simulink model "HEARTVI110"  (Simulink 5.0)
settings: Solver=ode45  StartTime=0.0  StopTime=3  RelTol=1e-3
libraries: simulink x3
settings Model: Creator=Dit Papa Lamine NDao  LastModifiedBy=formateur  SaveTime=off  SaveOutput=off  LimitDataPoints=off

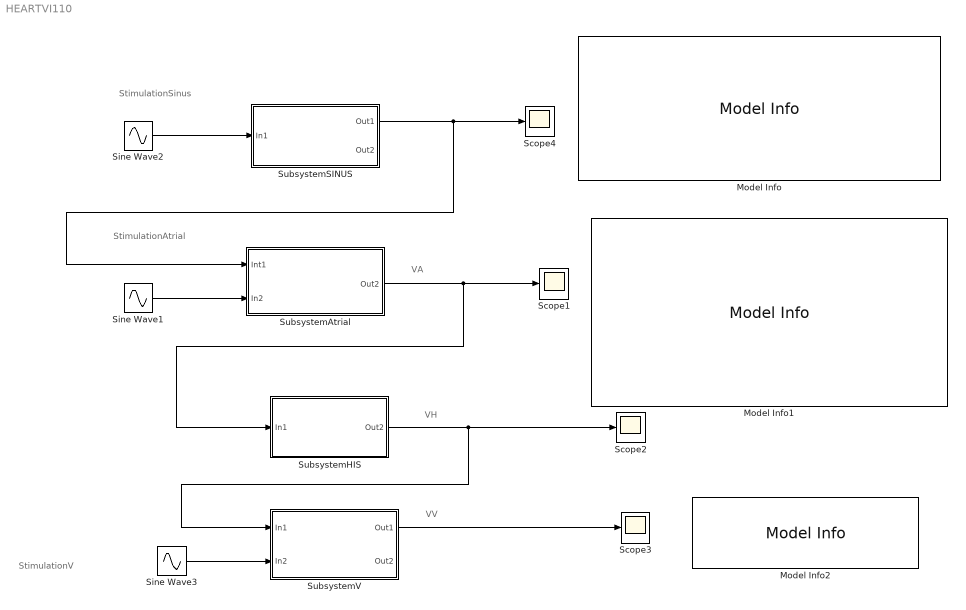
== system HEARTVI110 ==
  note: StimulationSinus
  note: StimulationAtrial
  note: VA
  note: VH
  note: VV
  note: StimulationV
  Model Info : simulink/Model-Wide Utilities/Model Info  InitialBlockCM=None  BlockCM=None  Frame=on  DisplayStringWithTags=|  HorizontalTextAlignment=Center  LeftAlignmentValue=0.5  SourceBlockDiagram=HEARTVI110  TagMaxNumber=20
      | NEW BLOCK LIBRARY SIMULINK
      | BLOCK HEART VI
      | TUTORIAL BY DIT.P.L.NDAO
      | BUREAU EA dakar senegal
      | www.cardiorythmor-vibrator.com
      | TUTORIAL N°1 date 8/12/2009
      | patants ndao france 2005
      | copyright ndao 2007
  Model Info1 : simulink/Model-Wide Utilities/Model Info  InitialBlockCM=None  BlockCM=None  Frame=on  DisplayStringWithTags=|  HorizontalTextAlignment=Center  LeftAlignmentValue=0.5  SourceBlockDiagram=HEARTVI110  TagMaxNumber=20
      | INVESTIGATION WITH HEART VI1
      | 1)I begin with no normal heart beating 
      | Fs=2Fa=2Fv
      | 2)i change parameter sinus and
      |  i publish annihilation of heart rythm past days.
      | 3)I Re-Synchronize the heart beat i
      | n this case.
      | of no normal heart beating.
      | Rational cardiac parameters.
      | Stimulation of normal sinus rythm of sinus,that 
      | induces Polymorphic Arrythmias like Wakenbach Syndrom-Sinusal Stimulation means Central
      | nervous reaction---Input stimulation Asinwt
      | A=2  w=2
  Model Info2 : simulink/Model-Wide Utilities/Model Info  InitialBlockCM=None  BlockCM=None  Frame=on  DisplayStringWithTags=|  HorizontalTextAlignment=Center  LeftAlignmentValue=0.5  SourceBlockDiagram=HEARTVI110  TagMaxNumber=20
      | DATE;7/01/2010
      | -Sinusal stimulation of a normal sinus rythm
      | -Duration of computing:4mn
  Scope{1..4} (4 alike) : Scope
      Scope1 settings: YMin=-2  YMax=2  SaveName=ScopeData3
      Scope2 settings: YMin=-2  YMax=2  SaveName=ScopeData4
      Scope3 settings: YMin=-2  YMax=2  SaveName=ScopeData5
      Scope4 settings: YMin=-2  YMax=2  SaveName=ScopeData2
  Sine Wave1 : Sin  Amplitude=0  SampleTime=0
  Sine Wave2 : Sin  Amplitude=-206  Frequency=5  SampleTime=0
  Sine Wave3 : Sin  Amplitude=0  Frequency=2.4  SampleTime=0
  SubsystemAtrial : Subsystem
  SubsystemHIS : Subsystem
  SubsystemSINUS : Subsystem
  SubsystemV : Subsystem
  wires:
  SubsystemAtrial/1(Out2) -> Scope1/1, SubsystemHIS/1(In1)
  SubsystemHIS/1(Out2) -> Scope2/1, SubsystemV/1(In1)
  SubsystemV/1(Out1) -> Scope3/1
  Sine Wave2/1 -> SubsystemSINUS/1(In1)
  Sine Wave1/1 -> SubsystemAtrial/2(In2)
  Sine Wave3/1 -> SubsystemV/2(In2)
  SubsystemSINUS/1(Out1) -> SubsystemAtrial/1(Int1), Scope4/1

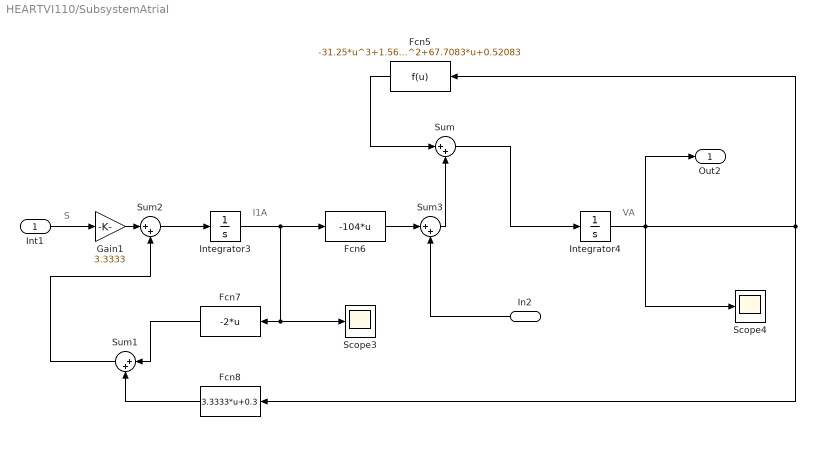
== system HEARTVI110/SubsystemAtrial ==
  note: I1A
  note: VA
  note: S
  Int1 : Inport  ShowAdditionalParam=on  DataType=double
  In2 : Inport  Orientation=left  Port=2
  Fcn5 : Fcn  Orientation=left  Expr=-31.25*u^3+1.5625*u^2+67.7083*u+0.52083
  Fcn6 : Fcn  Expr=-104*u
  Fcn7 : Fcn  Orientation=left  Expr=-2*u
  Fcn8 : Fcn  Orientation=left  Expr=3.3333*u+0.3
  Gain1 : Gain  Gain=3.3333  SaturateOnIntegerOverflow=on
  Integrator3 : Integrator  InitialCondition=0.00096  ZeroCross=off
  Integrator4 : Integrator  InitialCondition=-0.05  ZeroCross=off
  Scope3 : Scope
      settings: YMin=-2  YMax=2
  Scope4 : Scope
      settings: YMin=-2  YMax=2
  Sum : Sum  Inputs=|++  SaturateOnIntegerOverflow=on
  Sum1 : Sum  Orientation=left  Inputs=|++  SaturateOnIntegerOverflow=on
  Sum2 : Sum  Inputs=|++  SaturateOnIntegerOverflow=on
  Sum3 : Sum  Inputs=|++  SaturateOnIntegerOverflow=on
  Out2 : Outport
  wires:
  Fcn5/1 -> Sum/1
  Integrator3/1 -> Fcn6/1, Fcn7/1, Scope3/1
  Sum/1 -> Integrator4/1
  Integrator4/1 -> Fcn5/1, Fcn8/1, Scope4/1, Out2/1
  Fcn7/1 -> Sum1/1
  Fcn8/1 -> Sum1/2
  Fcn6/1 -> Sum3/1
  Sum3/1 -> Sum/2
  Int1/1 -> Gain1/1
  Gain1/1 -> Sum2/1
  Sum2/1 -> Integrator3/1
  Sum1/1 -> Sum2/2
  In2/1 -> Sum3/2

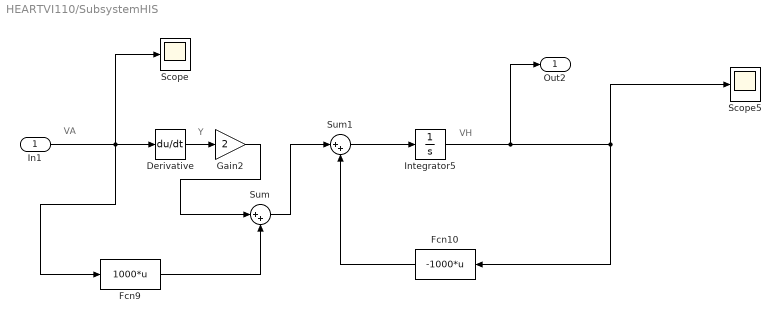
== system HEARTVI110/SubsystemHIS ==
  note: VH
  note: Y
  note: VA
  In1 : Inport  PortDimensions=159  ShowAdditionalParam=on  DataType=double
  Derivative : Derivative
  Fcn10 : Fcn  Orientation=left  Expr=-1000*u
  Fcn9 : Fcn  Expr=1000*u
  Gain2 : Gain  Gain=2  SaturateOnIntegerOverflow=on
  Integrator5 : Integrator  InitialCondition=-0.05  ZeroCross=off
  Scope : Scope
  Scope5 : Scope
      settings: YMin=-0.001  YMax=0.001
  Sum : Sum  Inputs=|++  SaturateOnIntegerOverflow=on
  Sum1 : Sum  Inputs=|++  SaturateOnIntegerOverflow=on
  Out2 : Outport
  wires:
  Integrator5/1 -> Fcn10/1, Scope5/1, Out2/1
  Fcn9/1 -> Sum/2
  Sum/1 -> Sum1/1
  Fcn10/1 -> Sum1/2
  Sum1/1 -> Integrator5/1
  Derivative/1 -> Gain2/1
  Gain2/1 -> Sum/1
  In1/1 -> Derivative/1, Scope/1, Fcn9/1

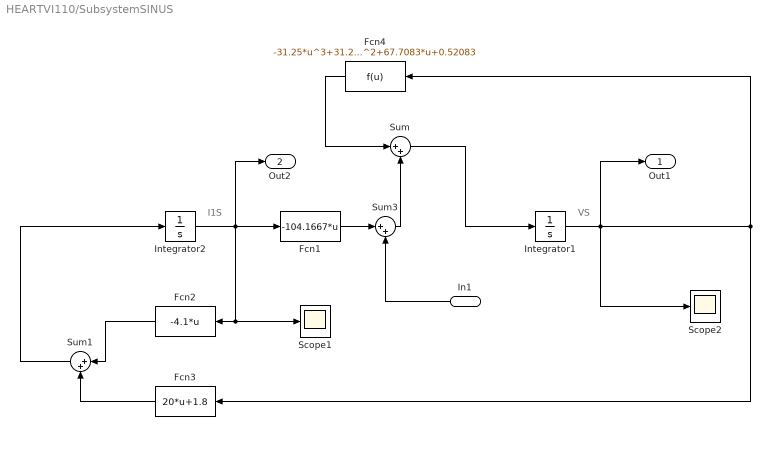
== system HEARTVI110/SubsystemSINUS ==
  note: I1S
  note: VS
  In1 : Inport  Orientation=left
  Fcn1 : Fcn  Expr=-104.1667*u
  Fcn2 : Fcn  Orientation=left  Expr=-4.1*u
  Fcn3 : Fcn  Orientation=left  Expr=20*u+1.8
  Fcn4 : Fcn  Orientation=left  Expr=-31.25*u^3+31.25*u^2+67.7083*u+0.52083
  Integrator1 : Integrator  InitialCondition=-0.05  ZeroCross=off
  Integrator2 : Integrator  InitialCondition=0.00096  ZeroCross=off
  Scope1 : Scope
      settings: YMin=-2  YMax=2
  Scope2 : Scope
      settings: YMin=-2  YMax=2
  Sum : Sum  Inputs=|++  SaturateOnIntegerOverflow=on
  Sum1 : Sum  Orientation=left  Inputs=|++  SaturateOnIntegerOverflow=on
  Sum3 : Sum  Inputs=|++  SaturateOnIntegerOverflow=on
  Out1 : Outport
  Out2 : Outport  Port=2
  wires:
  Fcn4/1 -> Sum/1
  Integrator2/1 -> Fcn1/1, Fcn2/1, Scope1/1, Out2/1
  Sum/1 -> Integrator1/1
  Integrator1/1 -> Fcn4/1, Fcn3/1, Scope2/1, Out1/1
  Fcn2/1 -> Sum1/1
  Fcn3/1 -> Sum1/2
  Fcn1/1 -> Sum3/1
  Sum3/1 -> Sum/2
  Sum1/1 -> Integrator2/1
  In1/1 -> Sum3/2

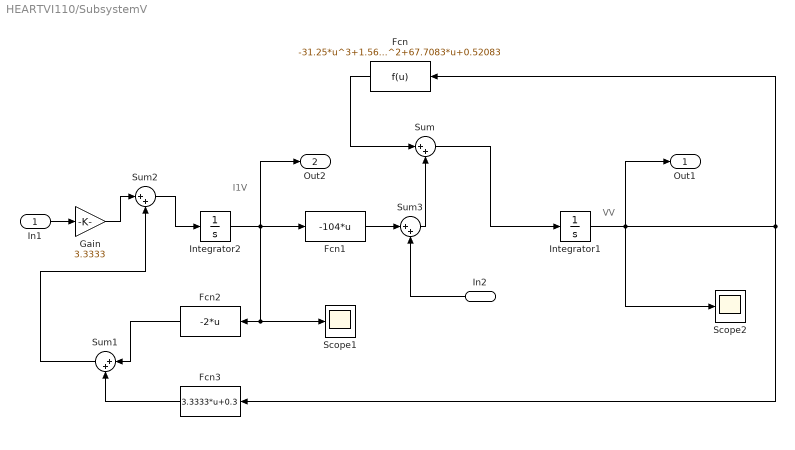
== system HEARTVI110/SubsystemV ==
  note: VV
  note: I1V
  In1 : Inport
  In2 : Inport  Orientation=left  Port=2
  Fcn : Fcn  Orientation=left  Expr=-31.25*u^3+1.5625*u^2+67.7083*u+0.52083
  Fcn1 : Fcn  Expr=-104*u
  Fcn2 : Fcn  Orientation=left  Expr=-2*u
  Fcn3 : Fcn  Orientation=left  Expr=3.3333*u+0.3
  Gain : Gain  Gain=3.3333  SaturateOnIntegerOverflow=on
  Integrator1 : Integrator  InitialCondition=-0.05  ZeroCross=off
  Integrator2 : Integrator  InitialCondition=0.00096  ZeroCross=off
  Scope1 : Scope
      settings: YMin=-2  YMax=2
  Scope2 : Scope
      settings: YMin=-2  YMax=2
  Sum : Sum  Inputs=|++  SaturateOnIntegerOverflow=on
  Sum1 : Sum  Orientation=left  Inputs=|++  SaturateOnIntegerOverflow=on
  Sum2 : Sum  Inputs=|++  SaturateOnIntegerOverflow=on
  Sum3 : Sum  Inputs=|++  SaturateOnIntegerOverflow=on
  Out1 : Outport
  Out2 : Outport  Port=2
  wires:
  In1/1 -> Gain/1
  In2/1 -> Sum3/2
  Sum1/1 -> Sum2/2
  Gain/1 -> Sum2/1
  Sum3/1 -> Sum/2
  Fcn1/1 -> Sum3/1
  Fcn3/1 -> Sum1/2
  Fcn2/1 -> Sum1/1
  Integrator1/1 -> Fcn/1, Fcn3/1, Out1/1, Scope2/1
  Sum/1 -> Integrator1/1
  Integrator2/1 -> Fcn1/1, Out2/1, Fcn2/1, Scope1/1
  Fcn/1 -> Sum/1
  Sum2/1 -> Integrator2/1
